simulink model "PID"  (R2025b)
settings: Solver=FixedStepAuto  StartTime=0.0  StopTime=1  RelTol=1e-3
InitFcn:
  | S = load("C:\Github\Tesis\src\matlab\Simulaciones Controladores\Desacople\DesacopleLin.mat","LinearAnalysisToolProject");
  | model = S.LinearAnalysisToolProject.Results(1).Data.Value;
  | A = model.A;
  | B = model.B;
  | C = model.C;
  | D = model.D;
  | 
  | Decimation_ADC = 64;     % Factor de decimación
  | Fs_ADC         = 3000;   % Frecuencia de muestreo de salida (Hz)
  | Vref           = 2.5;    % (V)
  | 
  | Ts_ADC = 1 / (Fs_ADC * Decimation_ADC);   % Período modulador (s)
  | Nyq    = Fs_ADC / 2;                       % Frecuencia de Nyquist (Hz)
  | Kpga = 50;
  | Kdirect = 2*Kpga;
  | Kinversa = -(Kpga-1);
values from neighbouring files (symbols this model uses):
  LinearAnalysisToolProject =     [DesacopleLin.mat]
undefined symbols (not defined in the file or in its folder): dspblkCoreblockFVToolHelper, gcbh
libraries: dspswit3 x1, slpidlib x1
settings Model: Creator=elias  LastModifiedBy=elias
settings OptimizationCC: DefaultParameterBehavior=Inlined  UseDivisionForNetSlopeComputation=on  GainParamInheritBuiltInType=on  UseFloatMulNetSlope=on  InlineInvariantSignals=on  EfficientFloat2IntCast=on  LifeSpan=1
settings DebuggingCC: AlgebraicLoopMsg=none
settings HardwareCC: ProdLongLongMode=on  TargetBitPerPointer=64.0  TargetBitPerSizeT=64.0  TargetBitPerPtrDiffT=64.0  TargetLongLongMode=on  TargetIntDivRoundTo=Zero  TargetEndianess=LittleEndian  TargetWordSize=64.0  TargetHWDeviceType=MATLAB Host  ProdEqTarget=off
settings SFSimCC: MATLABDynamicMemAlloc=off
settings RTWCC: SystemTargetFile=rsim.tlc  GenCodeOnly=on  TemplateMakefile=rsim_default_tmf  GenerateReport=on  Description=Rapid Simulation Target
settings CodeAppCC: ForceParamTrailComments=on
settings RSimTargetCC: ExtModeTransport=0.0  ExtModeStaticAllocSize=1000000.0  TargetLangStandard=C99 (ISO)  MultiwordLength=2048.0  DynamicStringBufferSize=256.0  CombineSignalStateStructs=on  MatFileLogging=off  PreserveMATLABNamespacesInGeneratedCode=on  SubcomponentCodeInterfacePackaging=Reusable function  SupportVariableSizeSignals=on  InstructionSetFMA=off  OptimizeReductions=off  LogToMDFFile=off

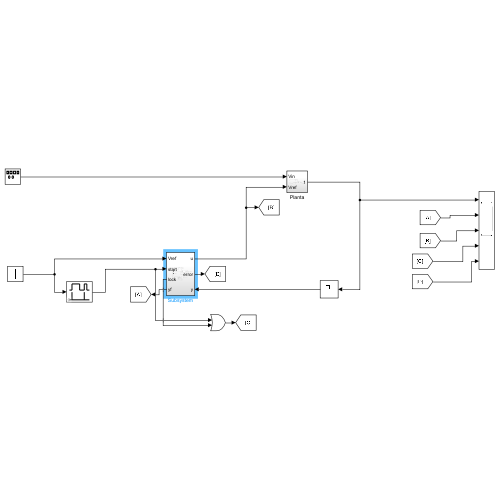
[thumbnail: Simulink's stored preview of the top-level diagram]
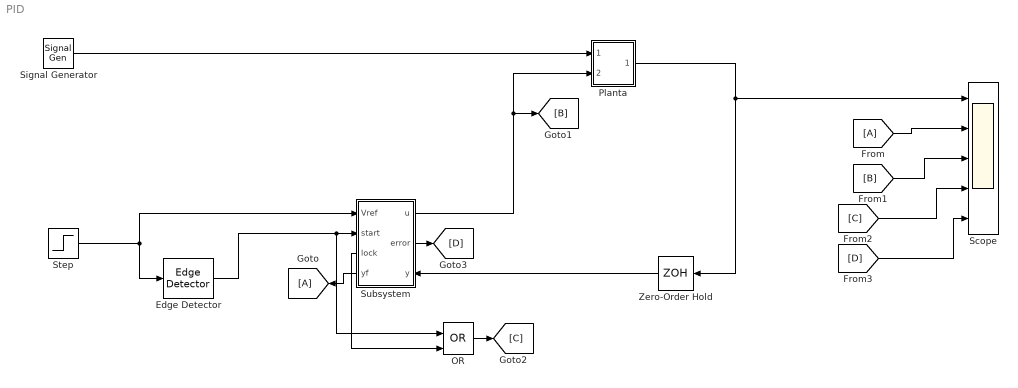
== system PID ==
  Edge Detector : dspswit3/Edge Detector
  From : From
  Goto : Goto
  OR : Logic  Operator=OR  IconShape=distinctive  AllPortsSameDT=off  OutDataTypeStr=boolean
  Planta : Subsystem
  Scope : Scope  NumInputPorts=5
      settings: ActiveDisplayYMinimum=-0.61485747802995938  ActiveDisplayYMaximum=4.5337977527076365
  Signal Generator : SignalGenerator  WaveForm=random  Amplitude=1e-3  Frequency=1/Fs_ADC
  Step : Step  Time=0.5  After=2.5  SampleTime=1/300
  Subsystem : Subsystem
      settings: PortSchema="{\"entries\":[{\"content\":{\"sides\":[{\"content\":{\"connectorIds\":[\"In1\",\"In2\",\"Out3\",\"Out4\"]},\"type\":\"ConnectorPlacement.EquallySpacedRectSide\",\"uuid\":\"38a9f17f-2329-4701-91c5-c4167a04ca54\"},{\"content\":{\"connectorIds\":[\"Out1\",\"Out2\",\"In3\"],\"side\":\"RIGHT\"},\"type\":\"ConnectorPlacement.EquallySpacedRectSide\",\"uuid\":\"2bfaa2de-a9fd-4df9-b0d2-09dc766593cb\"},{\"content\":{\"side\":\"TOP\"},\"type\":\"ConnectorPlacement.EquallySpacedRectSide\",\"uuid\":\"2307b6c3-8cb6-4080-9d98-8f294561747e\"}]},\"type\":\"ConnectorPlacement.EquallySpacedConnector\",\"uuid\":\"4a79aa29-1bb1-4a79-9b82-a1dd40bae461\"}],\"packageUris\":[\"http://schema.mathworks.com/mf0/Connector/R2020b\"],\"version\":\"1.0\"}"
  Zero-Order Hold : ZeroOrderHold  SampleTime=1/Fs_ADC
  wires:
  Step/1 -> Subsystem/1(Vref), Edge Detector/1
  Planta/1(Out1) -> Zero-Order Hold/1, Scope/1
  Signal Generator/1 -> Planta/1(Vin)
  Subsystem/1(u) -> Planta/2(Vref), [B]
  Zero-Order Hold/1 -> Subsystem/3(y)
  From/1 -> Scope/2
  [B] -> Scope/3
  Subsystem/4(yf) -> Goto/1
  Edge Detector/1 -> OR/1, Subsystem/2(start)
  [C] -> Scope/4
  Subsystem/2(error) -> [D]
  [D] -> Scope/5
  OR/1 -> [C]
  Subsystem/3(lock) -> OR/2

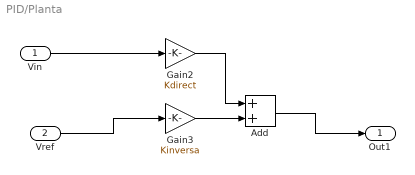
== system PID/Planta ==
  Vin : Inport
  Vref : Inport  Port=2
  Add : Sum
  Gain2 : Gain  Gain=Kdirect
  Gain3 : Gain  Gain=Kinversa
  Out1 : Outport
  wires:
  Gain2/1 -> Add/1
  Vref/1 -> Gain3/1
  Vin/1 -> Gain2/1
  Gain3/1 -> Add/2
  Add/1 -> Out1/1

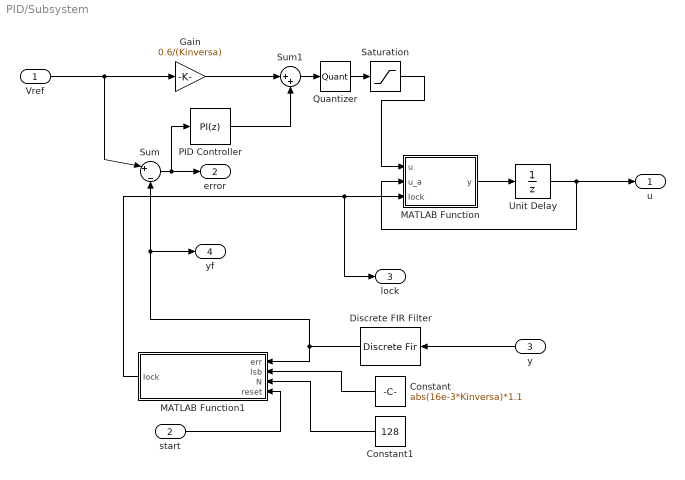
== system PID/Subsystem ==
  Vref : Inport
  start : Inport  Port=2
  y : Inport  Port=3
  Constant : Constant  Value=abs(16e-3*Kinversa)*1.1  SampleTime=1/3000
  Constant1 : Constant  Value=128
  Discrete FIR Filter : DiscreteFir  LoadFcn=dspblkCoreblockFVToolHelper(gcbh,'load');  Coefficients=fir1(127, 0.1/1500, hamming(127+1))
      settings: CopyFcn=dspblkCoreblockFVToolHelper(gcbh,'copy');  DeleteFcn=dspblkCoreblockFVToolHelper(gcbh,'close');  ModelCloseFcn=dspblkCoreblockFVToolHelper(gcbh,'close');  PreSaveFcn=dspblkCoreblockFVToolHelper(gcbh,'presave');  PostSaveFcn=dspblkCoreblockFVToolHelper(gcbh,'postsave');  CloseFcn=dspblkCoreblockFVToolHelper(gcbh,'close');
  Gain : Gain  Gain=0.6/(Kinversa)
  MATLAB Function : MATLAB Function  TreatAsAtomicUnit=on
  MATLAB Function1 : MATLAB Function  TreatAsAtomicUnit=on
  PID Controller : slpidlib/PID Controller  Controller=PI  Form=Parallel  TimeDomain=Discrete-time  UseExternalTs=off  SampleTime=-1  IntegratorMethod=Forward Euler  FilterMethod=Forward Euler  ControllerParametersSource=internal  P=-1e-3  I=-300e-6  UseKiTs=on  D=0  UseExternalDerivativeSource=off  N=100  UseFilter=on  TunerSelectOption=Transfer Function Based (PID Tuner App)  InitialConditionSource=internal  InitialConditionForIntegrator=0  InitialConditionForFilter=0  DifferentiatorICPrevScaledInput=0  ExternalReset=none  TrackingMode=off  Kt=1  LimitOutput=on  SatLimitsSource=internal  UpperSaturationLimit=4.08  LowerSaturationLimit=0  LinearizeAsGain=off  AntiWindupMode=clamping  Kb=1  LimitIntegrator=on  UpperIntegratorSaturationLimit=4.08  LowerIntegratorSaturationLimit=0  POutMin=[]  POutMax=[]  IOutMin=[]  IOutMax=[]  DOutMin=[]  DOutMax=[]  NOutMin=[]  NOutMax=[]  SumOutMin=[]  SumOutMax=[]  SaturationOutMin=[]  SaturationOutMax=[]  PParamMin=[]  PParamMax=[]  IParamMin=[]  IParamMax=[]  DParamMin=[]  DParamMax=[]  NParamMin=[]  NParamMax=[]  KbParamMin=[]  KbParamMax=[]  KtParamMin=[]  KtParamMax=[]  KbOutMin=[]  KbOutMax=[]  KtOutMin=[]  KtOutMax=[]  IntegratorOutMin=[]  IntegratorOutMax=[]  FilterOutMin=[]  FilterOutMax=[]  SumI1OutMin=[]  SumI1OutMax=[]  SumI2OutMin=[]  SumI2OutMax=[]  SumI3OutMin=[]  SumI3OutMax=[]  SumI4OutMin=[]  SumI4OutMax=[]  SumDOutMin=[]  SumDOutMax=[]  DifferentiatorOutMin=[]  DifferentiatorOutMax=[]  FilterDiffOutCoefMin=[]  FilterDiffOutCoefMax=[]  ReciprocalOutMin=[]  ReciprocalOutMax=[]  SumDenOutMin=[]  SumDenOutMax=[]  SumNumOutMin=[]  SumNumOutMax=[]  DivideOutMin=[]  DivideOutMax=[]  UdiffTsProdOutMin=[]  UdiffTsProdOutMax=[]  NTsProdOutMin=[]  NTsProdOutMax=[]  UintegralTsProdOutMin=[]  UintegralTsProdOutMax=[]  UngainTsProdOutMin=[]  UngainTsProdOutMax=[]  ClampingZeroOutDataTypeStr=Inherit: Inherit via back propagation  ClampingZeroOutMin=[]  ClampingZeroOutMax=[]  FilterDenConstantOutDataTypeStr=Inherit: Inherit via back propagation  FilterDenConstantOutMin=[]  FilterDenConstantOutMax=[]  PCopyOutDataTypeStr=Inherit: Inherit via back propagation  PCopyOutMin=[]  PCopyOutMax=[]  NCopyOutDataTypeStr=Inherit: Inherit via back propagation  NCopyOutMin=[]  NCopyOutMax=[]  IntegratorContinuousStateAttributes=''  IntegratorStateMustResolveToSignalObject=off  IntegratorRTWStateStorageClass=Auto  FilterContinuousStateAttributes=''  FilterStateMustResolveToSignalObject=off  FilterRTWStateStorageClass=Auto  ParallelPVariant=InternalParameters  IdealPVariant=Disabled  IVariant=InternalParameters  DVariant=Disabled  IntegratorVariant=Discrete  SatVariant=Enabled  AWVariant=DiscClampingParallel  PCopyVariant=Disabled  TRVariant=Disabled  FdbkBlocksVariant=Forward  IdealPFdbkVariant=Disabled  SatFdbkVariant=Disabled  DerivativeFilterVariant=Disabled  NVariant=Disabled  NCopyVariant=Disabled_SignalSpec  FilterICVariant=Disabled  IntegratorICVariant=InternalICs  ExternalResetVariant=Disabled  TRSumVariant=Passthrough  SumFdbkVariant=Disabled  SumVariant=Sum_PI  TsampFilterVariant=InternalTs  TsampNgainVariant=Passthrough  TsampIntegralVariant=Disabled_SignalSpec  ExternalSaturationOutDataTypeStr=Inherit: Same as second input  DerivativeSourceVariant=Disabled  PreIntVariant=InternalPreInt
  Quantizer : Quantizer  QuantizationInterval=16e-3
  Saturation : Saturate  UpperLimit=2.5  LowerLimit=-2.5
  Sum : Sum  Inputs=|+|-
  Sum1 : Sum  Inputs=|++
  Unit Delay : UnitDelay  SampleTime=-1  HasFrameUpgradeWarning=on
  u : Outport
  error : Outport  Port=2
  lock : Outport  Port=3
  yf : Outport  Port=4
  wires:
  PID Controller/1 -> Sum1/2
  Gain/1 -> Sum1/1
  Sum/1 -> error/1, PID Controller/1
  y/1 -> Discrete FIR Filter/1
  Vref/1 -> Sum/1, Gain/1
  MATLAB Function/1(y) -> Unit Delay/1
  Unit Delay/1 -> MATLAB Function/2(u_a), u/1
  Quantizer/1 -> Saturation/1
  Sum1/1 -> Quantizer/1
  Saturation/1 -> MATLAB Function/1(u)
  Discrete FIR Filter/1 -> yf/1, Sum/2, MATLAB Function1/1(err)
  Constant/1 -> MATLAB Function1/2(lsb)
  Constant1/1 -> MATLAB Function1/3(N)
  start/1 -> MATLAB Function1/4(reset)
  MATLAB Function1/1(lock) -> lock/1, MATLAB Function/3(lock)

== matlab function PID/Subsystem/MATLAB Function1 ==
  data: err input; lsb input; N input; reset input; lock output
function lock = detect_lock(err, lsb, N, reset)
%#codegen

persistent buf idx count locked

if isempty(buf)
    buf = zeros(1, N);
    idx = 1;
    count = 0;
    locked = false;
end

if reset
    buf(:) = 0;
    idx = 1;
    count = 0;
    locked = false;
    lock = false;
    return;
end

buf(idx) = err;

idx = idx + 1;
if idx > N
    idx = 1;
end

if count < N
    count = count + 1;
end

if count < N
    lock = false;
    return;
end

err_span = max(buf) - min(buf);

lock_threshold   = lsb;
unlock_threshold = 2*lsb;

if ~locked
    if err_span <= lock_threshold
        locked = true;
    end
else
    if err_span > unlock_threshold
        locked = false;
    end
end

lock = locked;

== matlab function PID/Subsystem/MATLAB Function ==
  data: u input; u_a input; lock input; y output
function y = fcn(u, u_a,lock)
    if lock == 1
        y = u_a;
    else
        y = u;
    end
end
